simulink model "Normal_Multiplier_M5_InXA2_NAB12"  (R2021a)
settings: Solver=VariableStepAuto  StartTime=0.0  StopTime=0.01  RelTol=1e-3
(part 1 of 2)
settings Model: SimulationMode=accelerator  Creator=PC  LastModifiedBy=PC

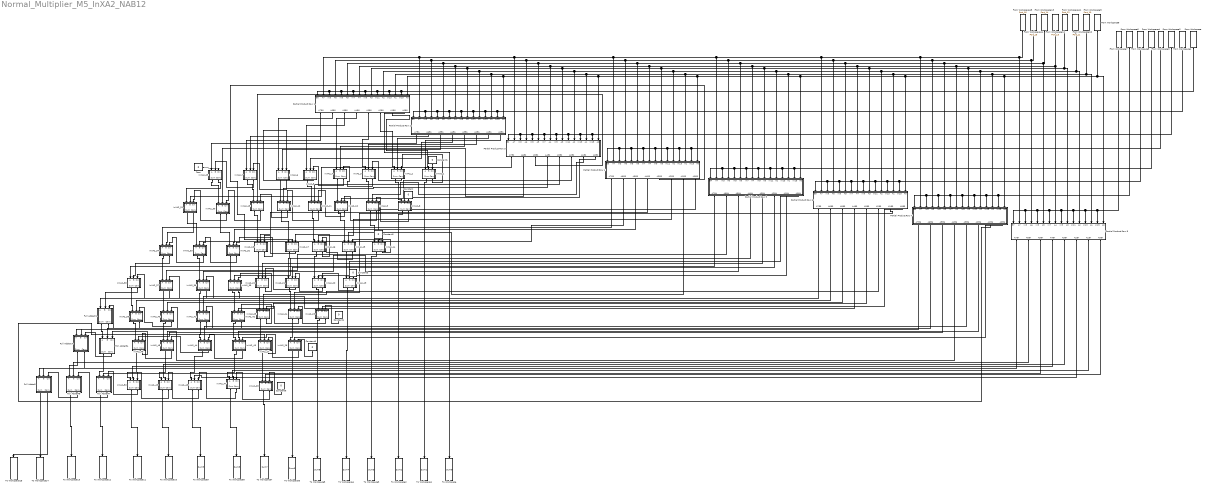
== system Normal_Multiplier_M5_InXA2_NAB12 ==
  Constant{,1..6} (7 alike) : Constant  Value=0
  From Workspace : FromWorkspace  VariableName=Port_1
  From Workspace1 : FromWorkspace  VariableName=Port_2
  From Workspace10 : FromWorkspace  VariableName=Port_11
  From Workspace11 : FromWorkspace  VariableName=Port_12
  From Workspace12 : FromWorkspace  VariableName=Port_13
  From Workspace13 : FromWorkspace  VariableName=Port_14
  From Workspace14 : FromWorkspace  VariableName=Port_15
  From Workspace15 : FromWorkspace  VariableName=Port_16
  From Workspace2 : FromWorkspace  VariableName=Port_3
  From Workspace3 : FromWorkspace  VariableName=Port_4
  From Workspace4 : FromWorkspace  VariableName=Port_5
  From Workspace5 : FromWorkspace  VariableName=Port_6
  From Workspace6 : FromWorkspace  VariableName=Port_7
  From Workspace7 : FromWorkspace  VariableName=Port_8
  From Workspace8 : FromWorkspace  VariableName=Port_9
  From Workspace9 : FromWorkspace  VariableName=Port_10
  Full Adder14 : Subsystem
  Full Adder21 : Subsystem
  Full Adder34 : Subsystem
  Full Adder47 : Subsystem
  Full Adder48 : Subsystem
  Full Adder5 : Subsystem
  InXA2_1 : Subsystem
  InXA2_10 : Subsystem
  InXA2_11 : Subsystem
  InXA2_12 : Subsystem
  InXA2_13 : Subsystem
  InXA2_14 : Subsystem
  InXA2_15 : Subsystem
  InXA2_16 : Subsystem
  InXA2_17 : Subsystem
  InXA2_18 : Subsystem
  InXA2_19 : Subsystem
  InXA2_2 : Subsystem
  InXA2_20 : Subsystem
  InXA2_21 : Subsystem
  InXA2_22 : Subsystem
  InXA2_23 : Subsystem
  InXA2_24 : Subsystem
  InXA2_25 : Subsystem
  InXA2_26 : Subsystem
  InXA2_27 : Subsystem
  InXA2_28 : Subsystem
  InXA2_29 : Subsystem
  InXA2_3 : Subsystem
  InXA2_30 : Subsystem
  InXA2_31 : Subsystem
  InXA2_32 : Subsystem
  InXA2_33 : Subsystem
  InXA2_34 : Subsystem
  InXA2_35 : Subsystem
  InXA2_36 : Subsystem
  InXA2_37 : Subsystem
  InXA2_38 : Subsystem
  InXA2_39 : Subsystem
  InXA2_4 : Subsystem
  InXA2_40 : Subsystem
  InXA2_41 : Subsystem
  InXA2_42 : Subsystem
  InXA2_43 : Subsystem
  InXA2_44 : Subsystem
  InXA2_45 : Subsystem
  InXA2_46 : Subsystem
  InXA2_47 : Subsystem
  InXA2_48 : Subsystem
  InXA2_49 : Subsystem
  InXA2_5 : Subsystem
  InXA2_50 : Subsystem
  InXA2_6 : Subsystem
  InXA2_7 : Subsystem
  InXA2_8 : Subsystem
  InXA2_9 : Subsystem
  Partial Product Row 1 : Subsystem
  Partial Product Row 2 : Subsystem
  Partial Product Row 3 : Subsystem
  Partial Product Row 4 : Subsystem
  Partial Product Row 5 : Subsystem
  Partial Product Row 6 : Subsystem
  Partial Product Row 7 : Subsystem
  Partial Product Row 8 : Subsystem
  To Workspace : ToWorkspace  VariableName=Sum0  SampleTime=0.01
      settings: Save2DSignal=2-D array (concatenate along first dimension)
  To Workspace1 : ToWorkspace  VariableName=Sum1  SampleTime=0.01
      settings: Save2DSignal=2-D array (concatenate along first dimension)
  To Workspace10 : ToWorkspace  VariableName=Sum10  SampleTime=0.01
      settings: Save2DSignal=2-D array (concatenate along first dimension)
  To Workspace11 : ToWorkspace  VariableName=Sum11  SampleTime=0.01
      settings: Save2DSignal=2-D array (concatenate along first dimension)
  To Workspace12 : ToWorkspace  VariableName=Sum12  SampleTime=0.01
      settings: Save2DSignal=2-D array (concatenate along first dimension)
  To Workspace13 : ToWorkspace  VariableName=Sum13  SampleTime=0.01
      settings: Save2DSignal=2-D array (concatenate along first dimension)
  To Workspace14 : ToWorkspace  VariableName=Sum14  SampleTime=0.01
      settings: Save2DSignal=2-D array (concatenate along first dimension)
  To Workspace15 : ToWorkspace  VariableName=Sum15  SampleTime=0.01
      settings: Save2DSignal=2-D array (concatenate along first dimension)
  To Workspace2 : ToWorkspace  VariableName=Sum2  SampleTime=0.01
      settings: Save2DSignal=2-D array (concatenate along first dimension)
  To Workspace3 : ToWorkspace  VariableName=Sum3  SampleTime=0.01
      settings: Save2DSignal=2-D array (concatenate along first dimension)
  To Workspace4 : ToWorkspace  VariableName=Sum4  SampleTime=0.01
      settings: Save2DSignal=2-D array (concatenate along first dimension)
  To Workspace5 : ToWorkspace  VariableName=Sum5  SampleTime=0.01
      settings: Save2DSignal=2-D array (concatenate along first dimension)
  To Workspace6 : ToWorkspace  VariableName=Sum6  SampleTime=0.01
      settings: Save2DSignal=2-D array (concatenate along first dimension)
  To Workspace7 : ToWorkspace  VariableName=Sum7  SampleTime=0.01
      settings: Save2DSignal=2-D array (concatenate along first dimension)
  To Workspace8 : ToWorkspace  VariableName=Sum8  SampleTime=0.01
      settings: Save2DSignal=2-D array (concatenate along first dimension)
  To Workspace9 : ToWorkspace  VariableName=Sum9  SampleTime=0.01
      settings: Save2DSignal=2-D array (concatenate along first dimension)
  Zero : Constant  Value=0  OutDataTypeStr=Inherit: Inherit via back propagation
  wires:
  Constant6/1 -> InXA2_28/3(Cin)
  InXA2_26/2(Carry) -> InXA2_27/3(Cin)
  Partial Product Row 6/7(A1B5) -> InXA2_24/2(B)
  Constant5/1 -> InXA2_26/3(Cin)
  Constant1/1 -> InXA2_1/3(Cin)
  Constant3/1 -> InXA2_19/3(Cin)
  InXA2_24/2(Carry) -> InXA2_25/3(Cin)
  Constant4/1 -> InXA2_23/3(Cin)
  Constant2/1 -> InXA2_14/3(Cin)
  InXA2_25/1(Sum) -> InXA2_27/1(A)
  Partial Product Row 8/2(A6B7) -> Full Adder48/2(B)
  Partial Product Row 5/8(A0B4) -> InXA2_19/2(B)
  InXA2_21/2(Carry) -> InXA2_22/3(Cin)
  InXA2_39/2(Carry) -> Full Adder21/3(Cin)
  InXA2_36/2(Carry) -> InXA2_37/3(Cin)
  Full Adder48/1(Sum) -> To Workspace13/1
  InXA2_7/2(Carry) -> InXA2_29/2(B)
  Full Adder14/1(Sum) -> Full Adder48/1(A)
  InXA2_9/1(Sum) -> InXA2_14/1(A)
  From Workspace7/1 -> Partial Product Row 8/11(In11), Partial Product Row 8/9(In9), Partial Product Row 8/7(In7), Partial Product Row 8/5(In5), Partial Product Row 8/3(In3), Partial Product Row 8/1(B7), Partial Product Row 8/13(In13), Partial Product Row 8/15(In15)
  Partial Product Row 7/3(A5B6) -> InXA2_46/2(B)
  Partial Product Row 8/4(A4B7) -> InXA2_50/2(B)
  Full Adder34/2(Carry) -> Full Adder14/3(Cin)
  InXA2_48/2(Carry) -> InXA2_49/3(Cin)
  Partial Product Row 8/6(A2B7) -> InXA2_48/2(B)
  Partial Product Row 7/7(A1B6) -> InXA2_27/2(B)
  InXA2_16/1(Sum) -> InXA2_20/1(A)
  Partial Product Row 8/7(A1B7) -> InXA2_47/2(B)
  Full Adder5/2(Carry) -> To Workspace15/1
  Partial Product Row 8/1(A7B7) -> Full Adder5/1(A)
  From Workspace4/1 -> Partial Product Row 5/15(In15), Partial Product Row 5/13(In13), Partial Product Row 5/11(In11), Partial Product Row 5/7(In7), Partial Product Row 5/5(In5), Partial Product Row 5/1(B4), Partial Product Row 5/3(In3), Partial Product Row 5/9(In9)
  Constant/1 -> InXA2_8/3(Cin)
  InXA2_36/1(Sum) -> InXA2_41/1(A)
  InXA2_38/2(Carry) -> Full Adder21/2(B)
  InXA2_8/2(Carry) -> InXA2_9/3(Cin)
  InXA2_27/1(Sum) -> InXA2_28/1(A)
  InXA2_9/2(Carry) -> InXA2_10/3(Cin)
  Full Adder48/2(Carry) -> Full Adder5/3(Cin)
  Full Adder47/1(Sum) -> To Workspace12/1
  InXA2_47/1(Sum) -> To Workspace8/1
  InXA2_5/1(Sum) -> InXA2_11/1(A)
  InXA2_49/1(Sum) -> To Workspace10/1
  InXA2_48/1(Sum) -> To Workspace9/1
  Partial Product Row 2/4(A4B1) -> InXA2_5/2(B)
  InXA2_39/1(Sum) -> InXA2_46/1(A)
  Partial Product Row 5/2(A6B4) -> InXA2_37/2(B)
  Partial Product Row 4/4(A4B3) -> InXA2_18/2(B)
  From Workspace3/1 -> Partial Product Row 4/15(In15), Partial Product Row 4/13(In13), Partial Product Row 4/11(In11), Partial Product Row 4/9(In9), Partial Product Row 4/7(In7), Partial Product Row 4/5(In5), Partial Product Row 4/1(B3), Partial Product Row 4/3(In3)
  Partial Product Row 7/1(A7B6) -> Full Adder14/1(A)
  InXA2_23/2(Carry) -> InXA2_24/3(Cin)
  Partial Product Row 7/4(A4B6) -> InXA2_45/2(B)
  Partial Product Row 6/1(A7B5) -> Full Adder21/1(A)
  Partial Product Row 8/3(A5B7) -> Full Adder47/2(B)
  Partial Product Row 7/2(A6B6) -> Full Adder34/2(B)
  Partial Product Row 7/6(A2B6) -> InXA2_43/2(B)
  Partial Product Row 3/6(A2B2) -> InXA2_10/2(B)
  InXA2_28/1(Sum) -> To Workspace7/1
  InXA2_15/2(Carry) -> InXA2_16/3(Cin)
  From Workspace13/1 -> Partial Product Row 8/6(A5), Partial Product Row 6/6(A5), Partial Product Row 4/6(A5), Partial Product Row 3/6(A5), Partial Product Row 1/6(A5), Partial Product Row 2/6(A5), Partial Product Row 5/6(A5), Partial Product Row 7/6(A5)
  InXA2_20/1(Sum) -> InXA2_23/1(A)
  Partial Product Row 2/8(A0B1) -> InXA2_1/1(A)
  InXA2_35/1(Sum) -> InXA2_42/1(A)
  InXA2_44/2(Carry) -> InXA2_45/3(Cin)
  InXA2_25/2(Carry) -> InXA2_42/3(Cin)
  InXA2_45/2(Carry) -> InXA2_46/3(Cin)
  InXA2_35/2(Carry) -> InXA2_36/3(Cin)
  InXA2_42/2(Carry) -> InXA2_41/3(Cin)
  Partial Product Row 2/3(A5B1) -> InXA2_6/2(B)
  Partial Product Row 3/8(A0B2) -> InXA2_8/2(B)
  Partial Product Row 7/8(A0B6) -> InXA2_26/2(B)
  Partial Product Row 2/2(A6B1) -> InXA2_7/2(B)
  From Workspace10/1 -> Partial Product Row 8/12(A2), Partial Product Row 7/12(A2), Partial Product Row 5/12(A2), Partial Product Row 4/12(A2), Partial Product Row 3/12(A2), Partial Product Row 1/12(A2), Partial Product Row 2/12(A2), Partial Product Row 6/12(A2)
  InXA2_41/1(Sum) -> InXA2_44/1(A)
  Partial Product Row 6/2(A6B5) -> InXA2_39/2(B)
  Partial Product Row 5/4(A4B4) -> InXA2_35/2(B)
  InXA2_32/1(Sum) -> InXA2_35/1(A)
  InXA2_20/2(Carry) -> InXA2_21/3(Cin)
  Partial Product Row 6/4(A4B5) -> InXA2_41/2(B)
  InXA2_40/2(Carry) -> InXA2_39/3(Cin)
  Partial Product Row 3/3(A5B2) -> InXA2_13/2(B)
  Partial Product Row 5/3(A5B4) -> InXA2_36/2(B)
  InXA2_17/2(Carry) -> InXA2_18/3(Cin)
  Partial Product Row 6/5(A3B5) -> InXA2_42/2(B)
  Partial Product Row 6/8(A0B5) -> InXA2_23/2(B)
  Full Adder21/2(Carry) -> Full Adder14/2(B)
  Partial Product Row 5/1(A7B4) -> InXA2_38/1(A)
  Partial Product Row 3/4(A4B2) -> InXA2_12/2(B)
  InXA2_31/1(Sum) -> InXA2_33/1(A)
  InXA2_50/2(Carry) -> Full Adder47/3(Cin)
  InXA2_12/1(Sum) -> InXA2_17/1(A)
  Partial Product Row 4/1(A7B3) -> InXA2_34/1(A)
  Partial Product Row 3/1(A7B2) -> InXA2_31/2(B)
  InXA2_3/2(Carry) -> InXA2_4/3(Cin)
  Partial Product Row 3/5(A3B2) -> InXA2_11/2(B)
  Partial Product Row 4/5(A3B3) -> InXA2_17/2(B)
  Partial Product Row 4/8(A0B3) -> InXA2_14/2(B)
  Partial Product Row 5/7(A1B4) -> InXA2_20/2(B)
  Partial Product Row 1/3(A5B0) -> InXA2_5/1(A)
  InXA2_24/1(Sum) -> InXA2_26/1(A)
  InXA2_29/2(Carry) -> InXA2_31/1(A)
  Partial Product Row 1/8(A0B0) -> To Workspace/1
  InXA2_3/1(Sum) -> InXA2_9/1(A)
  InXA2_1/1(Sum) -> To Workspace1/1
  Full Adder21/1(Sum) -> Full Adder34/1(A)
  InXA2_10/1(Sum) -> InXA2_15/1(A)
  Full Adder5/1(Sum) -> To Workspace14/1
  InXA2_38/1(Sum) -> InXA2_39/1(A)
  InXA2_42/1(Sum) -> InXA2_43/1(A)
  InXA2_4/1(Sum) -> InXA2_10/1(A)
  From Workspace12/1 -> Partial Product Row 8/8(A4), Partial Product Row 6/8(A4), Partial Product Row 4/8(A4), Partial Product Row 3/8(A4), Partial Product Row 1/8(A4), Partial Product Row 2/8(A4), Partial Product Row 5/8(A4), Partial Product Row 7/8(A4)
  InXA2_29/1(Sum) -> InXA2_30/1(A)
  Full Adder34/1(Sum) -> Full Adder47/1(A)
  InXA2_40/1(Sum) -> InXA2_45/1(A)
  From Workspace14/1 -> Partial Product Row 8/4(A6), Partial Product Row 7/4(A6), Partial Product Row 6/4(A6), Partial Product Row 5/4(A6), Partial Product Row 4/4(A6), Partial Product Row 3/4(A6), Partial Product Row 1/4(A6), Partial Product Row 2/4(A6)
  Partial Product Row 4/6(A2B3) -> InXA2_16/2(B)
  From Workspace11/1 -> Partial Product Row 8/10(A3), Partial Product Row 6/10(A3), Partial Product Row 4/10(A3), Partial Product Row 3/10(A3), Partial Product Row 1/10(A3), Partial Product Row 2/10(A3), Partial Product Row 5/10(A3), Partial Product Row 7/10(A3)
  From Workspace9/1 -> Partial Product Row 8/14(A1), Partial Product Row 7/14(A1), Partial Product Row 4/14(A1), Partial Product Row 1/14(A1), Partial Product Row 2/14(A1), Partial Product Row 3/14(A1), Partial Product Row 5/14(A1), Partial Product Row 6/14(A1)
  Partial Product Row 4/3(A5B3) -> InXA2_32/2(B)
  InXA2_43/1(Sum) -> InXA2_47/1(A)
  InXA2_33/1(Sum) -> InXA2_36/1(A)
  Partial Product Row 7/5(A3B6) -> InXA2_44/2(B)
  InXA2_12/2(Carry) -> InXA2_13/3(Cin)
  Partial Product Row 5/6(A2B4) -> InXA2_21/2(B)
  Partial Product Row 1/2(A6B0) -> InXA2_6/1(A)
  InXA2_6/1(Sum) -> InXA2_12/1(A)
  InXA2_21/1(Sum) -> InXA2_24/1(A)
  InXA2_22/1(Sum) -> InXA2_25/1(A)
  InXA2_11/1(Sum) -> InXA2_16/1(A)
  InXA2_34/1(Sum) -> InXA2_37/1(A)
  InXA2_26/1(Sum) -> To Workspace6/1
  Partial Product Row 2/7(A1B1) -> InXA2_2/2(B)
  InXA2_37/2(Carry) -> InXA2_38/3(Cin)
  From Workspace8/1 -> Partial Product Row 8/16(A0), Partial Product Row 7/16(A0), Partial Product Row 6/16(A0), Partial Product Row 4/16(A0), Partial Product Row 3/16(A0), Partial Product Row 1/16(A0), Partial Product Row 2/16(A0), Partial Product Row 5/16(A0)
  InXA2_34/2(Carry) -> InXA2_38/2(B)
  InXA2_19/2(Carry) -> InXA2_20/3(Cin)
  InXA2_41/2(Carry) -> InXA2_40/3(Cin)
  InXA2_45/1(Sum) -> InXA2_49/1(A)
  Partial Product Row 6/3(A5B5) -> InXA2_40/2(B)
  InXA2_1/2(Carry) -> InXA2_2/3(Cin)
  Partial Product Row 4/2(A6B3) -> InXA2_33/2(B)
  From Workspace15/1 -> Partial Product Row 7/2(A7), Partial Product Row 5/2(A7), Partial Product Row 4/2(A7), Partial Product Row 3/2(A7), Partial Product Row 1/2(A7), Partial Product Row 2/2(A7), Partial Product Row 6/2(A7), Partial Product Row 8/2(A7)
  InXA2_13/1(Sum) -> InXA2_18/1(A)
  InXA2_8/1(Sum) -> To Workspace2/1
  Partial Product Row 4/7(A1B3) -> InXA2_15/2(B)
  InXA2_30/1(Sum) -> InXA2_32/1(A)
  InXA2_14/2(Carry) -> InXA2_15/3(Cin)
  From Workspace/1 -> Partial Product Row 1/3(In3), Partial Product Row 1/1(B0), Partial Product Row 1/5(In5), Partial Product Row 1/7(In7), Partial Product Row 1/9(In9), Partial Product Row 1/11(In11), Partial Product Row 1/13(In13), Partial Product Row 1/15(In15)
  InXA2_13/2(Carry) -> InXA2_30/3(Cin)
  InXA2_10/2(Carry) -> InXA2_11/3(Cin)
  Partial Product Row 2/6(A2B1) -> InXA2_3/2(B)
  InXA2_23/1(Sum) -> To Workspace5/1
  Partial Product Row 2/5(A3B1) -> InXA2_4/2(B)
  InXA2_5/2(Carry) -> InXA2_6/3(Cin)
  InXA2_19/1(Sum) -> To Workspace4/1
  InXA2_30/2(Carry) -> InXA2_31/3(Cin)
  Partial Product Row 8/5(A3B7) -> InXA2_49/2(B)
  InXA2_33/2(Carry) -> InXA2_34/3(Cin)
  InXA2_31/2(Carry) -> InXA2_34/2(B)
  InXA2_32/2(Carry) -> InXA2_33/3(Cin)
  Partial Product Row 1/5(A3B0) -> InXA2_3/1(A)
  Partial Product Row 1/6(A2B0) -> InXA2_2/1(A)
  Partial Product Row 8/8(A0B7) -> InXA2_28/2(B)
  Full Adder47/2(Carry) -> Full Adder48/3(Cin)
  InXA2_28/2(Carry) -> InXA2_47/3(Cin)
  InXA2_18/2(Carry) -> InXA2_32/3(Cin)
  Partial Product Row 1/1(A7B0) -> InXA2_7/1(A)
  InXA2_44/1(Sum) -> InXA2_48/1(A)
  InXA2_47/2(Carry) -> InXA2_48/3(Cin)
  Partial Product Row 3/2(A6B2) -> InXA2_30/2(B)
  InXA2_4/2(Carry) -> InXA2_5/3(Cin)
  InXA2_43/2(Carry) -> InXA2_44/3(Cin)
  InXA2_46/2(Carry) -> Full Adder34/3(Cin)
  InXA2_14/1(Sum) -> To Workspace3/1
  InXA2_15/1(Sum) -> InXA2_19/1(A)
  InXA2_2/1(Sum) -> InXA2_8/1(A)
  InXA2_46/1(Sum) -> InXA2_50/1(A)
  From Workspace5/1 -> Partial Product Row 6/7(In7), Partial Product Row 6/5(In5), Partial Product Row 6/1(B5), Partial Product Row 6/3(In3), Partial Product Row 6/9(In9), Partial Product Row 6/11(In11), Partial Product Row 6/13(In13), Partial Product Row 6/15(In15)
  Partial Product Row 6/6(A2B5) -> InXA2_25/2(B)
  InXA2_18/1(Sum) -> InXA2_22/1(A)
  InXA2_16/2(Carry) -> InXA2_17/3(Cin)
  Partial Product Row 2/1(A7B1) -> InXA2_29/1(A)
  Partial Product Row 3/7(A1B2) -> InXA2_9/2(B)
  InXA2_37/1(Sum) -> InXA2_40/1(A)
  Partial Product Row 1/4(A4B0) -> InXA2_4/1(A)
  InXA2_27/2(Carry) -> InXA2_43/3(Cin)
  Partial Product Row 1/7(A1B0) -> InXA2_1/2(B)
  InXA2_7/1(Sum) -> InXA2_13/1(A)
  From Workspace6/1 -> Partial Product Row 7/13(In13), Partial Product Row 7/7(In7), Partial Product Row 7/5(In5), Partial Product Row 7/1(B6), Partial Product Row 7/3(In3), Partial Product Row 7/9(In9), Partial Product Row 7/11(In11), Partial Product Row 7/15(In15)
  InXA2_17/1(Sum) -> InXA2_21/1(A)
  InXA2_22/2(Carry) -> InXA2_35/3(Cin)
  InXA2_6/2(Carry) -> InXA2_7/3(Cin)
  InXA2_11/2(Carry) -> InXA2_12/3(Cin)
  Full Adder14/2(Carry) -> Full Adder5/2(B)
  InXA2_49/2(Carry) -> InXA2_50/3(Cin)
  Partial Product Row 5/5(A3B4) -> InXA2_22/2(B)
  From Workspace2/1 -> Partial Product Row 3/13(In13), Partial Product Row 3/7(In7), Partial Product Row 3/5(In5), Partial Product Row 3/3(In3), Partial Product Row 3/1(B2), Partial Product Row 3/9(In9), Partial Product Row 3/11(In11), Partial Product Row 3/15(In15)
  InXA2_50/1(Sum) -> To Workspace11/1
  InXA2_2/2(Carry) -> InXA2_3/3(Cin)
  From Workspace1/1 -> Partial Product Row 2/15(In15), Partial Product Row 2/5(In5), Partial Product Row 2/3(In3), Partial Product Row 2/1(B1), Partial Product Row 2/7(In7), Partial Product Row 2/9(In9), Partial Product Row 2/11(In11), Partial Product Row 2/13(In13)
  Zero/1 -> InXA2_29/3(Cin)

== system Normal_Multiplier_M5_InXA2_NAB12/Full Adder14 ==
  A : Inport
  B : Inport  Port=2
  Cin : Inport  Port=3
  Half Adder : Subsystem
  Half Adder1 : Subsystem
  Logical Operator : Logic  Operator=OR  AllPortsSameDT=off  OutDataTypeStr=boolean
  Sum : Outport
  Carry : Outport  Port=2
  wires:
  Cin/1 -> Half Adder1/1(In)
  Half Adder1/2(Cout) -> Logical Operator/1
  Half Adder/1(Sum) -> Half Adder1/2(Cin)
  Half Adder1/1(Sum) -> Sum/1
  Half Adder/2(Cout) -> Logical Operator/2
  A/1 -> Half Adder/1(In)
  B/1 -> Half Adder/2(Cin)
  Logical Operator/1 -> Carry/1

== system Normal_Multiplier_M5_InXA2_NAB12/Full Adder21 ==
  A : Inport
  B : Inport  Port=2
  Cin : Inport  Port=3
  Half Adder : Subsystem
  Half Adder1 : Subsystem
  Logical Operator : Logic  Operator=OR  AllPortsSameDT=off  OutDataTypeStr=boolean
  Sum : Outport
  Carry : Outport  Port=2
  wires:
  Cin/1 -> Half Adder1/1(In)
  Half Adder1/2(Cout) -> Logical Operator/1
  Half Adder/1(Sum) -> Half Adder1/2(Cin)
  Half Adder1/1(Sum) -> Sum/1
  Half Adder/2(Cout) -> Logical Operator/2
  A/1 -> Half Adder/1(In)
  B/1 -> Half Adder/2(Cin)
  Logical Operator/1 -> Carry/1

== system Normal_Multiplier_M5_InXA2_NAB12/Full Adder34 ==
  A : Inport
  B : Inport  Port=2
  Cin : Inport  Port=3
  Half Adder : Subsystem
  Half Adder1 : Subsystem
  Logical Operator : Logic  Operator=OR  AllPortsSameDT=off  OutDataTypeStr=boolean
  Sum : Outport
  Carry : Outport  Port=2
  wires:
  Cin/1 -> Half Adder1/1(In)
  Half Adder1/2(Cout) -> Logical Operator/1
  Half Adder/1(Sum) -> Half Adder1/2(Cin)
  Half Adder1/1(Sum) -> Sum/1
  Half Adder/2(Cout) -> Logical Operator/2
  A/1 -> Half Adder/1(In)
  B/1 -> Half Adder/2(Cin)
  Logical Operator/1 -> Carry/1

== system Normal_Multiplier_M5_InXA2_NAB12/Full Adder47 ==
  A : Inport
  B : Inport  Port=2
  Cin : Inport  Port=3
  Half Adder : Subsystem
  Half Adder1 : Subsystem
  Logical Operator : Logic  Operator=OR  AllPortsSameDT=off  OutDataTypeStr=boolean
  Sum : Outport
  Carry : Outport  Port=2
  wires:
  Cin/1 -> Half Adder1/1(In)
  Half Adder1/2(Cout) -> Logical Operator/1
  Half Adder/1(Sum) -> Half Adder1/2(Cin)
  Half Adder1/1(Sum) -> Sum/1
  Half Adder/2(Cout) -> Logical Operator/2
  A/1 -> Half Adder/1(In)
  B/1 -> Half Adder/2(Cin)
  Logical Operator/1 -> Carry/1

== system Normal_Multiplier_M5_InXA2_NAB12/Full Adder48 ==
  A : Inport
  B : Inport  Port=2
  Cin : Inport  Port=3
  Half Adder : Subsystem
  Half Adder1 : Subsystem
  Logical Operator : Logic  Operator=OR  AllPortsSameDT=off  OutDataTypeStr=boolean
  Sum : Outport
  Carry : Outport  Port=2
  wires:
  Cin/1 -> Half Adder1/1(In)
  Half Adder1/2(Cout) -> Logical Operator/1
  Half Adder/1(Sum) -> Half Adder1/2(Cin)
  Half Adder1/1(Sum) -> Sum/1
  Half Adder/2(Cout) -> Logical Operator/2
  A/1 -> Half Adder/1(In)
  B/1 -> Half Adder/2(Cin)
  Logical Operator/1 -> Carry/1

== system Normal_Multiplier_M5_InXA2_NAB12/Full Adder5 ==
  A : Inport
  B : Inport  Port=2
  Cin : Inport  Port=3
  Half Adder : Subsystem
  Half Adder1 : Subsystem
  Logical Operator : Logic  Operator=OR  AllPortsSameDT=off  OutDataTypeStr=boolean
  Sum : Outport
  Carry : Outport  Port=2
  wires:
  Cin/1 -> Half Adder1/1(In)
  Half Adder1/2(Cout) -> Logical Operator/1
  Half Adder/1(Sum) -> Half Adder1/2(Cin)
  Half Adder1/1(Sum) -> Sum/1
  Half Adder/2(Cout) -> Logical Operator/2
  A/1 -> Half Adder/1(In)
  B/1 -> Half Adder/2(Cin)
  Logical Operator/1 -> Carry/1

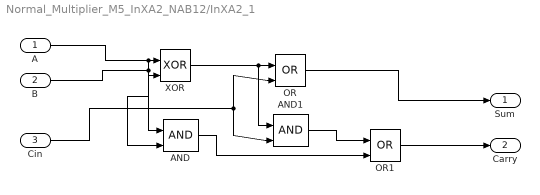
== system Normal_Multiplier_M5_InXA2_NAB12/InXA2_1 ==
  A : Inport
  B : Inport  Port=2
  Cin : Inport  Port=3
  AND : Logic  IconShape=distinctive  AllPortsSameDT=off  OutDataTypeStr=boolean
  AND1 : Logic  IconShape=distinctive  AllPortsSameDT=off  OutDataTypeStr=boolean
  OR : Logic  Operator=OR  IconShape=distinctive  AllPortsSameDT=off  OutDataTypeStr=boolean
  OR1 : Logic  Operator=OR  IconShape=distinctive  AllPortsSameDT=off  OutDataTypeStr=boolean
  XOR : Logic  Operator=XOR  IconShape=distinctive  AllPortsSameDT=off  OutDataTypeStr=boolean
  Sum : Outport
  Carry : Outport  Port=2
  wires:
  A/1 -> AND/1, XOR/1
  B/1 -> AND/2, XOR/2
  Cin/1 -> AND1/2, OR/2
  XOR/1 -> AND1/1, OR/1
  AND1/1 -> OR1/1
  AND/1 -> OR1/2
  OR1/1 -> Carry/1
  OR/1 -> Sum/1

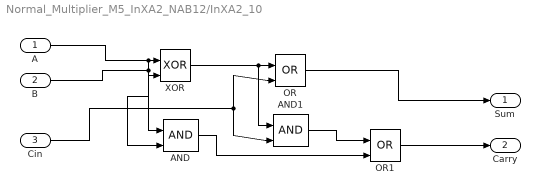
== system Normal_Multiplier_M5_InXA2_NAB12/InXA2_10 ==
  A : Inport
  B : Inport  Port=2
  Cin : Inport  Port=3
  AND : Logic  IconShape=distinctive  AllPortsSameDT=off  OutDataTypeStr=boolean
  AND1 : Logic  IconShape=distinctive  AllPortsSameDT=off  OutDataTypeStr=boolean
  OR : Logic  Operator=OR  IconShape=distinctive  AllPortsSameDT=off  OutDataTypeStr=boolean
  OR1 : Logic  Operator=OR  IconShape=distinctive  AllPortsSameDT=off  OutDataTypeStr=boolean
  XOR : Logic  Operator=XOR  IconShape=distinctive  AllPortsSameDT=off  OutDataTypeStr=boolean
  Sum : Outport
  Carry : Outport  Port=2
  wires:
  A/1 -> AND/1, XOR/1
  B/1 -> AND/2, XOR/2
  Cin/1 -> AND1/2, OR/2
  XOR/1 -> AND1/1, OR/1
  AND1/1 -> OR1/1
  AND/1 -> OR1/2
  OR1/1 -> Carry/1
  OR/1 -> Sum/1

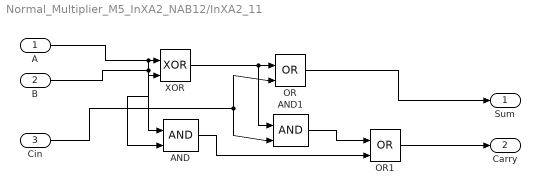
== system Normal_Multiplier_M5_InXA2_NAB12/InXA2_11 ==
  A : Inport
  B : Inport  Port=2
  Cin : Inport  Port=3
  AND : Logic  IconShape=distinctive  AllPortsSameDT=off  OutDataTypeStr=boolean
  AND1 : Logic  IconShape=distinctive  AllPortsSameDT=off  OutDataTypeStr=boolean
  OR : Logic  Operator=OR  IconShape=distinctive  AllPortsSameDT=off  OutDataTypeStr=boolean
  OR1 : Logic  Operator=OR  IconShape=distinctive  AllPortsSameDT=off  OutDataTypeStr=boolean
  XOR : Logic  Operator=XOR  IconShape=distinctive  AllPortsSameDT=off  OutDataTypeStr=boolean
  Sum : Outport
  Carry : Outport  Port=2
  wires:
  A/1 -> AND/1, XOR/1
  B/1 -> AND/2, XOR/2
  Cin/1 -> AND1/2, OR/2
  XOR/1 -> AND1/1, OR/1
  AND1/1 -> OR1/1
  AND/1 -> OR1/2
  OR1/1 -> Carry/1
  OR/1 -> Sum/1

== system Normal_Multiplier_M5_InXA2_NAB12/InXA2_12 ==
  A : Inport
  B : Inport  Port=2
  Cin : Inport  Port=3
  AND : Logic  IconShape=distinctive  AllPortsSameDT=off  OutDataTypeStr=boolean
  AND1 : Logic  IconShape=distinctive  AllPortsSameDT=off  OutDataTypeStr=boolean
  OR : Logic  Operator=OR  IconShape=distinctive  AllPortsSameDT=off  OutDataTypeStr=boolean
  OR1 : Logic  Operator=OR  IconShape=distinctive  AllPortsSameDT=off  OutDataTypeStr=boolean
  XOR : Logic  Operator=XOR  IconShape=distinctive  AllPortsSameDT=off  OutDataTypeStr=boolean
  Sum : Outport
  Carry : Outport  Port=2
  wires:
  A/1 -> AND/1, XOR/1
  B/1 -> AND/2, XOR/2
  Cin/1 -> AND1/2, OR/2
  XOR/1 -> AND1/1, OR/1
  AND1/1 -> OR1/1
  AND/1 -> OR1/2
  OR1/1 -> Carry/1
  OR/1 -> Sum/1

== system Normal_Multiplier_M5_InXA2_NAB12/InXA2_13 ==
  A : Inport
  B : Inport  Port=2
  Cin : Inport  Port=3
  AND : Logic  IconShape=distinctive  AllPortsSameDT=off  OutDataTypeStr=boolean
  AND1 : Logic  IconShape=distinctive  AllPortsSameDT=off  OutDataTypeStr=boolean
  OR : Logic  Operator=OR  IconShape=distinctive  AllPortsSameDT=off  OutDataTypeStr=boolean
  OR1 : Logic  Operator=OR  IconShape=distinctive  AllPortsSameDT=off  OutDataTypeStr=boolean
  XOR : Logic  Operator=XOR  IconShape=distinctive  AllPortsSameDT=off  OutDataTypeStr=boolean
  Sum : Outport
  Carry : Outport  Port=2
  wires:
  A/1 -> AND/1, XOR/1
  B/1 -> AND/2, XOR/2
  Cin/1 -> AND1/2, OR/2
  XOR/1 -> AND1/1, OR/1
  AND1/1 -> OR1/1
  AND/1 -> OR1/2
  OR1/1 -> Carry/1
  OR/1 -> Sum/1

== system Normal_Multiplier_M5_InXA2_NAB12/InXA2_14 ==
  A : Inport
  B : Inport  Port=2
  Cin : Inport  Port=3
  AND : Logic  IconShape=distinctive  AllPortsSameDT=off  OutDataTypeStr=boolean
  AND1 : Logic  IconShape=distinctive  AllPortsSameDT=off  OutDataTypeStr=boolean
  OR : Logic  Operator=OR  IconShape=distinctive  AllPortsSameDT=off  OutDataTypeStr=boolean
  OR1 : Logic  Operator=OR  IconShape=distinctive  AllPortsSameDT=off  OutDataTypeStr=boolean
  XOR : Logic  Operator=XOR  IconShape=distinctive  AllPortsSameDT=off  OutDataTypeStr=boolean
  Sum : Outport
  Carry : Outport  Port=2
  wires:
  A/1 -> AND/1, XOR/1
  B/1 -> AND/2, XOR/2
  Cin/1 -> AND1/2, OR/2
  XOR/1 -> AND1/1, OR/1
  AND1/1 -> OR1/1
  AND/1 -> OR1/2
  OR1/1 -> Carry/1
  OR/1 -> Sum/1

== system Normal_Multiplier_M5_InXA2_NAB12/InXA2_15 ==
  A : Inport
  B : Inport  Port=2
  Cin : Inport  Port=3
  AND : Logic  IconShape=distinctive  AllPortsSameDT=off  OutDataTypeStr=boolean
  AND1 : Logic  IconShape=distinctive  AllPortsSameDT=off  OutDataTypeStr=boolean
  OR : Logic  Operator=OR  IconShape=distinctive  AllPortsSameDT=off  OutDataTypeStr=boolean
  OR1 : Logic  Operator=OR  IconShape=distinctive  AllPortsSameDT=off  OutDataTypeStr=boolean
  XOR : Logic  Operator=XOR  IconShape=distinctive  AllPortsSameDT=off  OutDataTypeStr=boolean
  Sum : Outport
  Carry : Outport  Port=2
  wires:
  A/1 -> AND/1, XOR/1
  B/1 -> AND/2, XOR/2
  Cin/1 -> AND1/2, OR/2
  XOR/1 -> AND1/1, OR/1
  AND1/1 -> OR1/1
  AND/1 -> OR1/2
  OR1/1 -> Carry/1
  OR/1 -> Sum/1

== system Normal_Multiplier_M5_InXA2_NAB12/InXA2_16 ==
  A : Inport
  B : Inport  Port=2
  Cin : Inport  Port=3
  AND : Logic  IconShape=distinctive  AllPortsSameDT=off  OutDataTypeStr=boolean
  AND1 : Logic  IconShape=distinctive  AllPortsSameDT=off  OutDataTypeStr=boolean
  OR : Logic  Operator=OR  IconShape=distinctive  AllPortsSameDT=off  OutDataTypeStr=boolean
  OR1 : Logic  Operator=OR  IconShape=distinctive  AllPortsSameDT=off  OutDataTypeStr=boolean
  XOR : Logic  Operator=XOR  IconShape=distinctive  AllPortsSameDT=off  OutDataTypeStr=boolean
  Sum : Outport
  Carry : Outport  Port=2
  wires:
  A/1 -> AND/1, XOR/1
  B/1 -> AND/2, XOR/2
  Cin/1 -> AND1/2, OR/2
  XOR/1 -> AND1/1, OR/1
  AND1/1 -> OR1/1
  AND/1 -> OR1/2
  OR1/1 -> Carry/1
  OR/1 -> Sum/1

== system Normal_Multiplier_M5_InXA2_NAB12/InXA2_17 ==
  A : Inport
  B : Inport  Port=2
  Cin : Inport  Port=3
  AND : Logic  IconShape=distinctive  AllPortsSameDT=off  OutDataTypeStr=boolean
  AND1 : Logic  IconShape=distinctive  AllPortsSameDT=off  OutDataTypeStr=boolean
  OR : Logic  Operator=OR  IconShape=distinctive  AllPortsSameDT=off  OutDataTypeStr=boolean
  OR1 : Logic  Operator=OR  IconShape=distinctive  AllPortsSameDT=off  OutDataTypeStr=boolean
  XOR : Logic  Operator=XOR  IconShape=distinctive  AllPortsSameDT=off  OutDataTypeStr=boolean
  Sum : Outport
  Carry : Outport  Port=2
  wires:
  A/1 -> AND/1, XOR/1
  B/1 -> AND/2, XOR/2
  Cin/1 -> AND1/2, OR/2
  XOR/1 -> AND1/1, OR/1
  AND1/1 -> OR1/1
  AND/1 -> OR1/2
  OR1/1 -> Carry/1
  OR/1 -> Sum/1

== system Normal_Multiplier_M5_InXA2_NAB12/InXA2_18 ==
  A : Inport
  B : Inport  Port=2
  Cin : Inport  Port=3
  AND : Logic  IconShape=distinctive  AllPortsSameDT=off  OutDataTypeStr=boolean
  AND1 : Logic  IconShape=distinctive  AllPortsSameDT=off  OutDataTypeStr=boolean
  OR : Logic  Operator=OR  IconShape=distinctive  AllPortsSameDT=off  OutDataTypeStr=boolean
  OR1 : Logic  Operator=OR  IconShape=distinctive  AllPortsSameDT=off  OutDataTypeStr=boolean
  XOR : Logic  Operator=XOR  IconShape=distinctive  AllPortsSameDT=off  OutDataTypeStr=boolean
  Sum : Outport
  Carry : Outport  Port=2
  wires:
  A/1 -> AND/1, XOR/1
  B/1 -> AND/2, XOR/2
  Cin/1 -> AND1/2, OR/2
  XOR/1 -> AND1/1, OR/1
  AND1/1 -> OR1/1
  AND/1 -> OR1/2
  OR1/1 -> Carry/1
  OR/1 -> Sum/1

== system Normal_Multiplier_M5_InXA2_NAB12/InXA2_19 ==
  A : Inport
  B : Inport  Port=2
  Cin : Inport  Port=3
  AND : Logic  IconShape=distinctive  AllPortsSameDT=off  OutDataTypeStr=boolean
  AND1 : Logic  IconShape=distinctive  AllPortsSameDT=off  OutDataTypeStr=boolean
  OR : Logic  Operator=OR  IconShape=distinctive  AllPortsSameDT=off  OutDataTypeStr=boolean
  OR1 : Logic  Operator=OR  IconShape=distinctive  AllPortsSameDT=off  OutDataTypeStr=boolean
  XOR : Logic  Operator=XOR  IconShape=distinctive  AllPortsSameDT=off  OutDataTypeStr=boolean
  Sum : Outport
  Carry : Outport  Port=2
  wires:
  A/1 -> AND/1, XOR/1
  B/1 -> AND/2, XOR/2
  Cin/1 -> AND1/2, OR/2
  XOR/1 -> AND1/1, OR/1
  AND1/1 -> OR1/1
  AND/1 -> OR1/2
  OR1/1 -> Carry/1
  OR/1 -> Sum/1

== system Normal_Multiplier_M5_InXA2_NAB12/InXA2_2 ==
  A : Inport
  B : Inport  Port=2
  Cin : Inport  Port=3
  AND : Logic  IconShape=distinctive  AllPortsSameDT=off  OutDataTypeStr=boolean
  AND1 : Logic  IconShape=distinctive  AllPortsSameDT=off  OutDataTypeStr=boolean
  OR : Logic  Operator=OR  IconShape=distinctive  AllPortsSameDT=off  OutDataTypeStr=boolean
  OR1 : Logic  Operator=OR  IconShape=distinctive  AllPortsSameDT=off  OutDataTypeStr=boolean
  XOR : Logic  Operator=XOR  IconShape=distinctive  AllPortsSameDT=off  OutDataTypeStr=boolean
  Sum : Outport
  Carry : Outport  Port=2
  wires:
  A/1 -> AND/1, XOR/1
  B/1 -> AND/2, XOR/2
  Cin/1 -> AND1/2, OR/2
  XOR/1 -> AND1/1, OR/1
  AND1/1 -> OR1/1
  AND/1 -> OR1/2
  OR1/1 -> Carry/1
  OR/1 -> Sum/1

== system Normal_Multiplier_M5_InXA2_NAB12/InXA2_20 ==
  A : Inport
  B : Inport  Port=2
  Cin : Inport  Port=3
  AND : Logic  IconShape=distinctive  AllPortsSameDT=off  OutDataTypeStr=boolean
  AND1 : Logic  IconShape=distinctive  AllPortsSameDT=off  OutDataTypeStr=boolean
  OR : Logic  Operator=OR  IconShape=distinctive  AllPortsSameDT=off  OutDataTypeStr=boolean
  OR1 : Logic  Operator=OR  IconShape=distinctive  AllPortsSameDT=off  OutDataTypeStr=boolean
  XOR : Logic  Operator=XOR  IconShape=distinctive  AllPortsSameDT=off  OutDataTypeStr=boolean
  Sum : Outport
  Carry : Outport  Port=2
  wires:
  A/1 -> AND/1, XOR/1
  B/1 -> AND/2, XOR/2
  Cin/1 -> AND1/2, OR/2
  XOR/1 -> AND1/1, OR/1
  AND1/1 -> OR1/1
  AND/1 -> OR1/2
  OR1/1 -> Carry/1
  OR/1 -> Sum/1

== system Normal_Multiplier_M5_InXA2_NAB12/InXA2_21 ==
  A : Inport
  B : Inport  Port=2
  Cin : Inport  Port=3
  AND : Logic  IconShape=distinctive  AllPortsSameDT=off  OutDataTypeStr=boolean
  AND1 : Logic  IconShape=distinctive  AllPortsSameDT=off  OutDataTypeStr=boolean
  OR : Logic  Operator=OR  IconShape=distinctive  AllPortsSameDT=off  OutDataTypeStr=boolean
  OR1 : Logic  Operator=OR  IconShape=distinctive  AllPortsSameDT=off  OutDataTypeStr=boolean
  XOR : Logic  Operator=XOR  IconShape=distinctive  AllPortsSameDT=off  OutDataTypeStr=boolean
  Sum : Outport
  Carry : Outport  Port=2
  wires:
  A/1 -> AND/1, XOR/1
  B/1 -> AND/2, XOR/2
  Cin/1 -> AND1/2, OR/2
  XOR/1 -> AND1/1, OR/1
  AND1/1 -> OR1/1
  AND/1 -> OR1/2
  OR1/1 -> Carry/1
  OR/1 -> Sum/1

== system Normal_Multiplier_M5_InXA2_NAB12/InXA2_22 ==
  A : Inport
  B : Inport  Port=2
  Cin : Inport  Port=3
  AND : Logic  IconShape=distinctive  AllPortsSameDT=off  OutDataTypeStr=boolean
  AND1 : Logic  IconShape=distinctive  AllPortsSameDT=off  OutDataTypeStr=boolean
  OR : Logic  Operator=OR  IconShape=distinctive  AllPortsSameDT=off  OutDataTypeStr=boolean
  OR1 : Logic  Operator=OR  IconShape=distinctive  AllPortsSameDT=off  OutDataTypeStr=boolean
  XOR : Logic  Operator=XOR  IconShape=distinctive  AllPortsSameDT=off  OutDataTypeStr=boolean
  Sum : Outport
  Carry : Outport  Port=2
  wires:
  A/1 -> AND/1, XOR/1
  B/1 -> AND/2, XOR/2
  Cin/1 -> AND1/2, OR/2
  XOR/1 -> AND1/1, OR/1
  AND1/1 -> OR1/1
  AND/1 -> OR1/2
  OR1/1 -> Carry/1
  OR/1 -> Sum/1

== system Normal_Multiplier_M5_InXA2_NAB12/InXA2_23 ==
  A : Inport
  B : Inport  Port=2
  Cin : Inport  Port=3
  AND : Logic  IconShape=distinctive  AllPortsSameDT=off  OutDataTypeStr=boolean
  AND1 : Logic  IconShape=distinctive  AllPortsSameDT=off  OutDataTypeStr=boolean
  OR : Logic  Operator=OR  IconShape=distinctive  AllPortsSameDT=off  OutDataTypeStr=boolean
  OR1 : Logic  Operator=OR  IconShape=distinctive  AllPortsSameDT=off  OutDataTypeStr=boolean
  XOR : Logic  Operator=XOR  IconShape=distinctive  AllPortsSameDT=off  OutDataTypeStr=boolean
  Sum : Outport
  Carry : Outport  Port=2
  wires:
  A/1 -> AND/1, XOR/1
  B/1 -> AND/2, XOR/2
  Cin/1 -> AND1/2, OR/2
  XOR/1 -> AND1/1, OR/1
  AND1/1 -> OR1/1
  AND/1 -> OR1/2
  OR1/1 -> Carry/1
  OR/1 -> Sum/1

== system Normal_Multiplier_M5_InXA2_NAB12/InXA2_24 ==
  A : Inport
  B : Inport  Port=2
  Cin : Inport  Port=3
  AND : Logic  IconShape=distinctive  AllPortsSameDT=off  OutDataTypeStr=boolean
  AND1 : Logic  IconShape=distinctive  AllPortsSameDT=off  OutDataTypeStr=boolean
  OR : Logic  Operator=OR  IconShape=distinctive  AllPortsSameDT=off  OutDataTypeStr=boolean
  OR1 : Logic  Operator=OR  IconShape=distinctive  AllPortsSameDT=off  OutDataTypeStr=boolean
  XOR : Logic  Operator=XOR  IconShape=distinctive  AllPortsSameDT=off  OutDataTypeStr=boolean
  Sum : Outport
  Carry : Outport  Port=2
  wires:
  A/1 -> AND/1, XOR/1
  B/1 -> AND/2, XOR/2
  Cin/1 -> AND1/2, OR/2
  XOR/1 -> AND1/1, OR/1
  AND1/1 -> OR1/1
  AND/1 -> OR1/2
  OR1/1 -> Carry/1
  OR/1 -> Sum/1

== system Normal_Multiplier_M5_InXA2_NAB12/InXA2_25 ==
  A : Inport
  B : Inport  Port=2
  Cin : Inport  Port=3
  AND : Logic  IconShape=distinctive  AllPortsSameDT=off  OutDataTypeStr=boolean
  AND1 : Logic  IconShape=distinctive  AllPortsSameDT=off  OutDataTypeStr=boolean
  OR : Logic  Operator=OR  IconShape=distinctive  AllPortsSameDT=off  OutDataTypeStr=boolean
  OR1 : Logic  Operator=OR  IconShape=distinctive  AllPortsSameDT=off  OutDataTypeStr=boolean
  XOR : Logic  Operator=XOR  IconShape=distinctive  AllPortsSameDT=off  OutDataTypeStr=boolean
  Sum : Outport
  Carry : Outport  Port=2
  wires:
  A/1 -> AND/1, XOR/1
  B/1 -> AND/2, XOR/2
  Cin/1 -> AND1/2, OR/2
  XOR/1 -> AND1/1, OR/1
  AND1/1 -> OR1/1
  AND/1 -> OR1/2
  OR1/1 -> Carry/1
  OR/1 -> Sum/1

== system Normal_Multiplier_M5_InXA2_NAB12/InXA2_26 ==
  A : Inport
  B : Inport  Port=2
  Cin : Inport  Port=3
  AND : Logic  IconShape=distinctive  AllPortsSameDT=off  OutDataTypeStr=boolean
  AND1 : Logic  IconShape=distinctive  AllPortsSameDT=off  OutDataTypeStr=boolean
  OR : Logic  Operator=OR  IconShape=distinctive  AllPortsSameDT=off  OutDataTypeStr=boolean
  OR1 : Logic  Operator=OR  IconShape=distinctive  AllPortsSameDT=off  OutDataTypeStr=boolean
  XOR : Logic  Operator=XOR  IconShape=distinctive  AllPortsSameDT=off  OutDataTypeStr=boolean
  Sum : Outport
  Carry : Outport  Port=2
  wires:
  A/1 -> AND/1, XOR/1
  B/1 -> AND/2, XOR/2
  Cin/1 -> AND1/2, OR/2
  XOR/1 -> AND1/1, OR/1
  AND1/1 -> OR1/1
  AND/1 -> OR1/2
  OR1/1 -> Carry/1
  OR/1 -> Sum/1

== system Normal_Multiplier_M5_InXA2_NAB12/InXA2_27 ==
  A : Inport
  B : Inport  Port=2
  Cin : Inport  Port=3
  AND : Logic  IconShape=distinctive  AllPortsSameDT=off  OutDataTypeStr=boolean
  AND1 : Logic  IconShape=distinctive  AllPortsSameDT=off  OutDataTypeStr=boolean
  OR : Logic  Operator=OR  IconShape=distinctive  AllPortsSameDT=off  OutDataTypeStr=boolean
  OR1 : Logic  Operator=OR  IconShape=distinctive  AllPortsSameDT=off  OutDataTypeStr=boolean
  XOR : Logic  Operator=XOR  IconShape=distinctive  AllPortsSameDT=off  OutDataTypeStr=boolean
  Sum : Outport
  Carry : Outport  Port=2
  wires:
  A/1 -> AND/1, XOR/1
  B/1 -> AND/2, XOR/2
  Cin/1 -> AND1/2, OR/2
  XOR/1 -> AND1/1, OR/1
  AND1/1 -> OR1/1
  AND/1 -> OR1/2
  OR1/1 -> Carry/1
  OR/1 -> Sum/1

== system Normal_Multiplier_M5_InXA2_NAB12/InXA2_28 ==
  A : Inport
  B : Inport  Port=2
  Cin : Inport  Port=3
  AND : Logic  IconShape=distinctive  AllPortsSameDT=off  OutDataTypeStr=boolean
  AND1 : Logic  IconShape=distinctive  AllPortsSameDT=off  OutDataTypeStr=boolean
  OR : Logic  Operator=OR  IconShape=distinctive  AllPortsSameDT=off  OutDataTypeStr=boolean
  OR1 : Logic  Operator=OR  IconShape=distinctive  AllPortsSameDT=off  OutDataTypeStr=boolean
  XOR : Logic  Operator=XOR  IconShape=distinctive  AllPortsSameDT=off  OutDataTypeStr=boolean
  Sum : Outport
  Carry : Outport  Port=2
  wires:
  A/1 -> AND/1, XOR/1
  B/1 -> AND/2, XOR/2
  Cin/1 -> AND1/2, OR/2
  XOR/1 -> AND1/1, OR/1
  AND1/1 -> OR1/1
  AND/1 -> OR1/2
  OR1/1 -> Carry/1
  OR/1 -> Sum/1

== system Normal_Multiplier_M5_InXA2_NAB12/InXA2_29 ==
  A : Inport
  B : Inport  Port=2
  Cin : Inport  Port=3
  AND : Logic  IconShape=distinctive  AllPortsSameDT=off  OutDataTypeStr=boolean
  AND1 : Logic  IconShape=distinctive  AllPortsSameDT=off  OutDataTypeStr=boolean
  OR : Logic  Operator=OR  IconShape=distinctive  AllPortsSameDT=off  OutDataTypeStr=boolean
  OR1 : Logic  Operator=OR  IconShape=distinctive  AllPortsSameDT=off  OutDataTypeStr=boolean
  XOR : Logic  Operator=XOR  IconShape=distinctive  AllPortsSameDT=off  OutDataTypeStr=boolean
  Sum : Outport
  Carry : Outport  Port=2
  wires:
  A/1 -> AND/1, XOR/1
  B/1 -> AND/2, XOR/2
  Cin/1 -> AND1/2, OR/2
  XOR/1 -> AND1/1, OR/1
  AND1/1 -> OR1/1
  AND/1 -> OR1/2
  OR1/1 -> Carry/1
  OR/1 -> Sum/1

== system Normal_Multiplier_M5_InXA2_NAB12/InXA2_3 ==
  A : Inport
  B : Inport  Port=2
  Cin : Inport  Port=3
  AND : Logic  IconShape=distinctive  AllPortsSameDT=off  OutDataTypeStr=boolean
  AND1 : Logic  IconShape=distinctive  AllPortsSameDT=off  OutDataTypeStr=boolean
  OR : Logic  Operator=OR  IconShape=distinctive  AllPortsSameDT=off  OutDataTypeStr=boolean
  OR1 : Logic  Operator=OR  IconShape=distinctive  AllPortsSameDT=off  OutDataTypeStr=boolean
  XOR : Logic  Operator=XOR  IconShape=distinctive  AllPortsSameDT=off  OutDataTypeStr=boolean
  Sum : Outport
  Carry : Outport  Port=2
  wires:
  A/1 -> AND/1, XOR/1
  B/1 -> AND/2, XOR/2
  Cin/1 -> AND1/2, OR/2
  XOR/1 -> AND1/1, OR/1
  AND1/1 -> OR1/1
  AND/1 -> OR1/2
  OR1/1 -> Carry/1
  OR/1 -> Sum/1

== system Normal_Multiplier_M5_InXA2_NAB12/InXA2_30 ==
  A : Inport
  B : Inport  Port=2
  Cin : Inport  Port=3
  AND : Logic  IconShape=distinctive  AllPortsSameDT=off  OutDataTypeStr=boolean
  AND1 : Logic  IconShape=distinctive  AllPortsSameDT=off  OutDataTypeStr=boolean
  OR : Logic  Operator=OR  IconShape=distinctive  AllPortsSameDT=off  OutDataTypeStr=boolean
  OR1 : Logic  Operator=OR  IconShape=distinctive  AllPortsSameDT=off  OutDataTypeStr=boolean
  XOR : Logic  Operator=XOR  IconShape=distinctive  AllPortsSameDT=off  OutDataTypeStr=boolean
  Sum : Outport
  Carry : Outport  Port=2
  wires:
  A/1 -> AND/1, XOR/1
  B/1 -> AND/2, XOR/2
  Cin/1 -> AND1/2, OR/2
  XOR/1 -> AND1/1, OR/1
  AND1/1 -> OR1/1
  AND/1 -> OR1/2
  OR1/1 -> Carry/1
  OR/1 -> Sum/1

== system Normal_Multiplier_M5_InXA2_NAB12/InXA2_31 ==
  A : Inport
  B : Inport  Port=2
  Cin : Inport  Port=3
  AND : Logic  IconShape=distinctive  AllPortsSameDT=off  OutDataTypeStr=boolean
  AND1 : Logic  IconShape=distinctive  AllPortsSameDT=off  OutDataTypeStr=boolean
  OR : Logic  Operator=OR  IconShape=distinctive  AllPortsSameDT=off  OutDataTypeStr=boolean
  OR1 : Logic  Operator=OR  IconShape=distinctive  AllPortsSameDT=off  OutDataTypeStr=boolean
  XOR : Logic  Operator=XOR  IconShape=distinctive  AllPortsSameDT=off  OutDataTypeStr=boolean
  Sum : Outport
  Carry : Outport  Port=2
  wires:
  A/1 -> AND/1, XOR/1
  B/1 -> AND/2, XOR/2
  Cin/1 -> AND1/2, OR/2
  XOR/1 -> AND1/1, OR/1
  AND1/1 -> OR1/1
  AND/1 -> OR1/2
  OR1/1 -> Carry/1
  OR/1 -> Sum/1

== system Normal_Multiplier_M5_InXA2_NAB12/InXA2_32 ==
  A : Inport
  B : Inport  Port=2
  Cin : Inport  Port=3
  AND : Logic  IconShape=distinctive  AllPortsSameDT=off  OutDataTypeStr=boolean
  AND1 : Logic  IconShape=distinctive  AllPortsSameDT=off  OutDataTypeStr=boolean
  OR : Logic  Operator=OR  IconShape=distinctive  AllPortsSameDT=off  OutDataTypeStr=boolean
  OR1 : Logic  Operator=OR  IconShape=distinctive  AllPortsSameDT=off  OutDataTypeStr=boolean
  XOR : Logic  Operator=XOR  IconShape=distinctive  AllPortsSameDT=off  OutDataTypeStr=boolean
  Sum : Outport
  Carry : Outport  Port=2
  wires:
  A/1 -> AND/1, XOR/1
  B/1 -> AND/2, XOR/2
  Cin/1 -> AND1/2, OR/2
  XOR/1 -> AND1/1, OR/1
  AND1/1 -> OR1/1
  AND/1 -> OR1/2
  OR1/1 -> Carry/1
  OR/1 -> Sum/1

== system Normal_Multiplier_M5_InXA2_NAB12/InXA2_33 ==
  A : Inport
  B : Inport  Port=2
  Cin : Inport  Port=3
  AND : Logic  IconShape=distinctive  AllPortsSameDT=off  OutDataTypeStr=boolean
  AND1 : Logic  IconShape=distinctive  AllPortsSameDT=off  OutDataTypeStr=boolean
  OR : Logic  Operator=OR  IconShape=distinctive  AllPortsSameDT=off  OutDataTypeStr=boolean
  OR1 : Logic  Operator=OR  IconShape=distinctive  AllPortsSameDT=off  OutDataTypeStr=boolean
  XOR : Logic  Operator=XOR  IconShape=distinctive  AllPortsSameDT=off  OutDataTypeStr=boolean
  Sum : Outport
  Carry : Outport  Port=2
  wires:
  A/1 -> AND/1, XOR/1
  B/1 -> AND/2, XOR/2
  Cin/1 -> AND1/2, OR/2
  XOR/1 -> AND1/1, OR/1
  AND1/1 -> OR1/1
  AND/1 -> OR1/2
  OR1/1 -> Carry/1
  OR/1 -> Sum/1

== system Normal_Multiplier_M5_InXA2_NAB12/InXA2_34 ==
  A : Inport
  B : Inport  Port=2
  Cin : Inport  Port=3
  AND : Logic  IconShape=distinctive  AllPortsSameDT=off  OutDataTypeStr=boolean
  AND1 : Logic  IconShape=distinctive  AllPortsSameDT=off  OutDataTypeStr=boolean
  OR : Logic  Operator=OR  IconShape=distinctive  AllPortsSameDT=off  OutDataTypeStr=boolean
  OR1 : Logic  Operator=OR  IconShape=distinctive  AllPortsSameDT=off  OutDataTypeStr=boolean
  XOR : Logic  Operator=XOR  IconShape=distinctive  AllPortsSameDT=off  OutDataTypeStr=boolean
  Sum : Outport
  Carry : Outport  Port=2
  wires:
  A/1 -> AND/1, XOR/1
  B/1 -> AND/2, XOR/2
  Cin/1 -> AND1/2, OR/2
  XOR/1 -> AND1/1, OR/1
  AND1/1 -> OR1/1
  AND/1 -> OR1/2
  OR1/1 -> Carry/1
  OR/1 -> Sum/1

== system Normal_Multiplier_M5_InXA2_NAB12/InXA2_35 ==
  A : Inport
  B : Inport  Port=2
  Cin : Inport  Port=3
  AND : Logic  IconShape=distinctive  AllPortsSameDT=off  OutDataTypeStr=boolean
  AND1 : Logic  IconShape=distinctive  AllPortsSameDT=off  OutDataTypeStr=boolean
  OR : Logic  Operator=OR  IconShape=distinctive  AllPortsSameDT=off  OutDataTypeStr=boolean
  OR1 : Logic  Operator=OR  IconShape=distinctive  AllPortsSameDT=off  OutDataTypeStr=boolean
  XOR : Logic  Operator=XOR  IconShape=distinctive  AllPortsSameDT=off  OutDataTypeStr=boolean
  Sum : Outport
  Carry : Outport  Port=2
  wires:
  A/1 -> AND/1, XOR/1
  B/1 -> AND/2, XOR/2
  Cin/1 -> AND1/2, OR/2
  XOR/1 -> AND1/1, OR/1
  AND1/1 -> OR1/1
  AND/1 -> OR1/2
  OR1/1 -> Carry/1
  OR/1 -> Sum/1

== system Normal_Multiplier_M5_InXA2_NAB12/InXA2_36 ==
  A : Inport
  B : Inport  Port=2
  Cin : Inport  Port=3
  AND : Logic  IconShape=distinctive  AllPortsSameDT=off  OutDataTypeStr=boolean
  AND1 : Logic  IconShape=distinctive  AllPortsSameDT=off  OutDataTypeStr=boolean
  OR : Logic  Operator=OR  IconShape=distinctive  AllPortsSameDT=off  OutDataTypeStr=boolean
  OR1 : Logic  Operator=OR  IconShape=distinctive  AllPortsSameDT=off  OutDataTypeStr=boolean
  XOR : Logic  Operator=XOR  IconShape=distinctive  AllPortsSameDT=off  OutDataTypeStr=boolean
  Sum : Outport
  Carry : Outport  Port=2
  wires:
  A/1 -> AND/1, XOR/1
  B/1 -> AND/2, XOR/2
  Cin/1 -> AND1/2, OR/2
  XOR/1 -> AND1/1, OR/1
  AND1/1 -> OR1/1
  AND/1 -> OR1/2
  OR1/1 -> Carry/1
  OR/1 -> Sum/1

== system Normal_Multiplier_M5_InXA2_NAB12/InXA2_37 ==
  A : Inport
  B : Inport  Port=2
  Cin : Inport  Port=3
  AND : Logic  IconShape=distinctive  AllPortsSameDT=off  OutDataTypeStr=boolean
  AND1 : Logic  IconShape=distinctive  AllPortsSameDT=off  OutDataTypeStr=boolean
  OR : Logic  Operator=OR  IconShape=distinctive  AllPortsSameDT=off  OutDataTypeStr=boolean
  OR1 : Logic  Operator=OR  IconShape=distinctive  AllPortsSameDT=off  OutDataTypeStr=boolean
  XOR : Logic  Operator=XOR  IconShape=distinctive  AllPortsSameDT=off  OutDataTypeStr=boolean
  Sum : Outport
  Carry : Outport  Port=2
  wires:
  A/1 -> AND/1, XOR/1
  B/1 -> AND/2, XOR/2
  Cin/1 -> AND1/2, OR/2
  XOR/1 -> AND1/1, OR/1
  AND1/1 -> OR1/1
  AND/1 -> OR1/2
  OR1/1 -> Carry/1
  OR/1 -> Sum/1

== system Normal_Multiplier_M5_InXA2_NAB12/InXA2_38 ==
  A : Inport
  B : Inport  Port=2
  Cin : Inport  Port=3
  AND : Logic  IconShape=distinctive  AllPortsSameDT=off  OutDataTypeStr=boolean
  AND1 : Logic  IconShape=distinctive  AllPortsSameDT=off  OutDataTypeStr=boolean
  OR : Logic  Operator=OR  IconShape=distinctive  AllPortsSameDT=off  OutDataTypeStr=boolean
  OR1 : Logic  Operator=OR  IconShape=distinctive  AllPortsSameDT=off  OutDataTypeStr=boolean
  XOR : Logic  Operator=XOR  IconShape=distinctive  AllPortsSameDT=off  OutDataTypeStr=boolean
  Sum : Outport
  Carry : Outport  Port=2
  wires:
  A/1 -> AND/1, XOR/1
  B/1 -> AND/2, XOR/2
  Cin/1 -> AND1/2, OR/2
  XOR/1 -> AND1/1, OR/1
  AND1/1 -> OR1/1
  AND/1 -> OR1/2
  OR1/1 -> Carry/1
  OR/1 -> Sum/1

== system Normal_Multiplier_M5_InXA2_NAB12/InXA2_39 ==
  A : Inport
  B : Inport  Port=2
  Cin : Inport  Port=3
  AND : Logic  IconShape=distinctive  AllPortsSameDT=off  OutDataTypeStr=boolean
  AND1 : Logic  IconShape=distinctive  AllPortsSameDT=off  OutDataTypeStr=boolean
  OR : Logic  Operator=OR  IconShape=distinctive  AllPortsSameDT=off  OutDataTypeStr=boolean
  OR1 : Logic  Operator=OR  IconShape=distinctive  AllPortsSameDT=off  OutDataTypeStr=boolean
  XOR : Logic  Operator=XOR  IconShape=distinctive  AllPortsSameDT=off  OutDataTypeStr=boolean
  Sum : Outport
  Carry : Outport  Port=2
  wires:
  A/1 -> AND/1, XOR/1
  B/1 -> AND/2, XOR/2
  Cin/1 -> AND1/2, OR/2
  XOR/1 -> AND1/1, OR/1
  AND1/1 -> OR1/1
  AND/1 -> OR1/2
  OR1/1 -> Carry/1
  OR/1 -> Sum/1

== system Normal_Multiplier_M5_InXA2_NAB12/InXA2_4 ==
  A : Inport
  B : Inport  Port=2
  Cin : Inport  Port=3
  AND : Logic  IconShape=distinctive  AllPortsSameDT=off  OutDataTypeStr=boolean
  AND1 : Logic  IconShape=distinctive  AllPortsSameDT=off  OutDataTypeStr=boolean
  OR : Logic  Operator=OR  IconShape=distinctive  AllPortsSameDT=off  OutDataTypeStr=boolean
  OR1 : Logic  Operator=OR  IconShape=distinctive  AllPortsSameDT=off  OutDataTypeStr=boolean
  XOR : Logic  Operator=XOR  IconShape=distinctive  AllPortsSameDT=off  OutDataTypeStr=boolean
  Sum : Outport
  Carry : Outport  Port=2
  wires:
  A/1 -> AND/1, XOR/1
  B/1 -> AND/2, XOR/2
  Cin/1 -> AND1/2, OR/2
  XOR/1 -> AND1/1, OR/1
  AND1/1 -> OR1/1
  AND/1 -> OR1/2
  OR1/1 -> Carry/1
  OR/1 -> Sum/1

== system Normal_Multiplier_M5_InXA2_NAB12/InXA2_40 ==
  A : Inport
  B : Inport  Port=2
  Cin : Inport  Port=3
  AND : Logic  IconShape=distinctive  AllPortsSameDT=off  OutDataTypeStr=boolean
  AND1 : Logic  IconShape=distinctive  AllPortsSameDT=off  OutDataTypeStr=boolean
  OR : Logic  Operator=OR  IconShape=distinctive  AllPortsSameDT=off  OutDataTypeStr=boolean
  OR1 : Logic  Operator=OR  IconShape=distinctive  AllPortsSameDT=off  OutDataTypeStr=boolean
  XOR : Logic  Operator=XOR  IconShape=distinctive  AllPortsSameDT=off  OutDataTypeStr=boolean
  Sum : Outport
  Carry : Outport  Port=2
  wires:
  A/1 -> AND/1, XOR/1
  B/1 -> AND/2, XOR/2
  Cin/1 -> AND1/2, OR/2
  XOR/1 -> AND1/1, OR/1
  AND1/1 -> OR1/1
  AND/1 -> OR1/2
  OR1/1 -> Carry/1
  OR/1 -> Sum/1

== system Normal_Multiplier_M5_InXA2_NAB12/InXA2_41 ==
  A : Inport
  B : Inport  Port=2
  Cin : Inport  Port=3
  AND : Logic  IconShape=distinctive  AllPortsSameDT=off  OutDataTypeStr=boolean
  AND1 : Logic  IconShape=distinctive  AllPortsSameDT=off  OutDataTypeStr=boolean
  OR : Logic  Operator=OR  IconShape=distinctive  AllPortsSameDT=off  OutDataTypeStr=boolean
  OR1 : Logic  Operator=OR  IconShape=distinctive  AllPortsSameDT=off  OutDataTypeStr=boolean
  XOR : Logic  Operator=XOR  IconShape=distinctive  AllPortsSameDT=off  OutDataTypeStr=boolean
  Sum : Outport
  Carry : Outport  Port=2
  wires:
  A/1 -> AND/1, XOR/1
  B/1 -> AND/2, XOR/2
  Cin/1 -> AND1/2, OR/2
  XOR/1 -> AND1/1, OR/1
  AND1/1 -> OR1/1
  AND/1 -> OR1/2
  OR1/1 -> Carry/1
  OR/1 -> Sum/1

== system Normal_Multiplier_M5_InXA2_NAB12/InXA2_42 ==
  A : Inport
  B : Inport  Port=2
  Cin : Inport  Port=3
  AND : Logic  IconShape=distinctive  AllPortsSameDT=off  OutDataTypeStr=boolean
  AND1 : Logic  IconShape=distinctive  AllPortsSameDT=off  OutDataTypeStr=boolean
  OR : Logic  Operator=OR  IconShape=distinctive  AllPortsSameDT=off  OutDataTypeStr=boolean
  OR1 : Logic  Operator=OR  IconShape=distinctive  AllPortsSameDT=off  OutDataTypeStr=boolean
  XOR : Logic  Operator=XOR  IconShape=distinctive  AllPortsSameDT=off  OutDataTypeStr=boolean
  Sum : Outport
  Carry : Outport  Port=2
  wires:
  A/1 -> AND/1, XOR/1
  B/1 -> AND/2, XOR/2
  Cin/1 -> AND1/2, OR/2
  XOR/1 -> AND1/1, OR/1
  AND1/1 -> OR1/1
  AND/1 -> OR1/2
  OR1/1 -> Carry/1
  OR/1 -> Sum/1

== system Normal_Multiplier_M5_InXA2_NAB12/InXA2_43 ==
  A : Inport
  B : Inport  Port=2
  Cin : Inport  Port=3
  AND : Logic  IconShape=distinctive  AllPortsSameDT=off  OutDataTypeStr=boolean
  AND1 : Logic  IconShape=distinctive  AllPortsSameDT=off  OutDataTypeStr=boolean
  OR : Logic  Operator=OR  IconShape=distinctive  AllPortsSameDT=off  OutDataTypeStr=boolean
  OR1 : Logic  Operator=OR  IconShape=distinctive  AllPortsSameDT=off  OutDataTypeStr=boolean
  XOR : Logic  Operator=XOR  IconShape=distinctive  AllPortsSameDT=off  OutDataTypeStr=boolean
  Sum : Outport
  Carry : Outport  Port=2
  wires:
  A/1 -> AND/1, XOR/1
  B/1 -> AND/2, XOR/2
  Cin/1 -> AND1/2, OR/2
  XOR/1 -> AND1/1, OR/1
  AND1/1 -> OR1/1
  AND/1 -> OR1/2
  OR1/1 -> Carry/1
  OR/1 -> Sum/1
